simulink model "simple"  (R2025b)
settings: Solver=VariableStepAuto  StartTime=0.0  StopTime=10.0  RelTol=1e-3
undefined symbols (not defined in the file or in its folder): qd, qdot_d

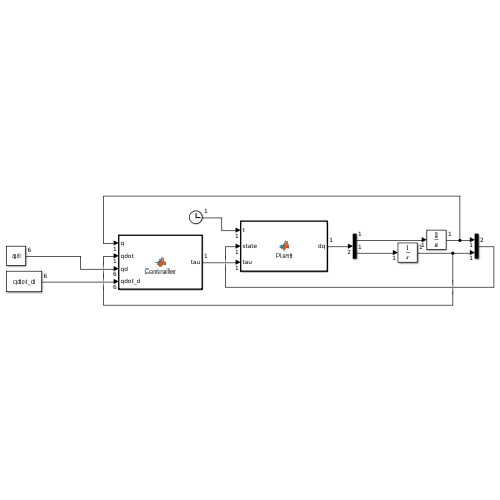
[thumbnail: Simulink's stored preview of the top-level diagram]
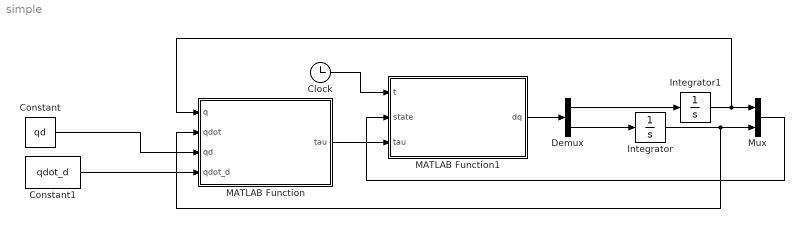
== system simple ==
  Clock : Clock
  Constant : Constant  Value=qd
  Constant1 : Constant  Value=qdot_d
  Demux : Demux  Outputs=2
  Integrator : Integrator
  Integrator1 : Integrator
  MATLAB Function : MATLAB Function  TreatAsAtomicUnit=on
  MATLAB Function1 : MATLAB Function  TreatAsAtomicUnit=on
  Mux : Mux  Inputs=2
  wires:
  Constant/1 -> MATLAB Function/3(qd)
  Constant1/1 -> MATLAB Function/4(qdot_d)
  MATLAB Function/1(tau) -> MATLAB Function1/3(tau)
  Integrator1/1 -> MATLAB Function/1(q), Mux/1
  Mux/1 -> MATLAB Function1/2(state)
  Clock/1 -> MATLAB Function1/1(t)
  MATLAB Function1/1(dq) -> Demux/1
  Demux/1 -> Integrator1/1
  Demux/2 -> Integrator/1
  Integrator/1 -> MATLAB Function/2(qdot), Mux/2

== matlab function simple/MATLAB Function1 ==
  data: t input; dq output; state input; tau input
function dq = Plant(t, state, tau)
    %#codegen
    dq = zeros(1, 12);
    persistent robot
    if isempty(robot)
        robot = robot_for_simulink();   % create robot ONCE
    end
   dq_internal = simpleUR5Plant(t, state, robot, tau);

   dq(1,:) = dq_internal;
end

== matlab function simple/MATLAB Function ==
  data: q input; tau output; qdot input; qd input; qdot_d input
function tau = Controller(q, qdot, qd, qdot_d)
tau = zeros(1, 6);

persistent robot
if isempty(robot)
    robot = robot_for_simulink();
end

tau_internal = simplePDControl(robot, q, qdot, qd, qdot_d);

tau(1,:) = tau_internal; 
end
